simulink model "TEST"  (R2021a)
settings: Solver=VariableStepAuto  StartTime=0.0  StopTime=10  RelTol=1e-3
undefined symbols (not defined in the file): f, Jw, Kb, Kt, La, Ra
libraries: vrlib x1
settings Model: Creator=mario  LastModifiedBy=mario
settings SolverCC: AlgebraicLoopSolver=TrustRegion
settings DataIOCC: ReturnWorkspaceOutputs=off
settings DebuggingCC: SFMachineParentedDataDiag=warning  ArithmeticOperatorsInVariantConditions=warning
settings SFSimCC: CustomCodeUndefinedFunction=UseInterfaceOnly

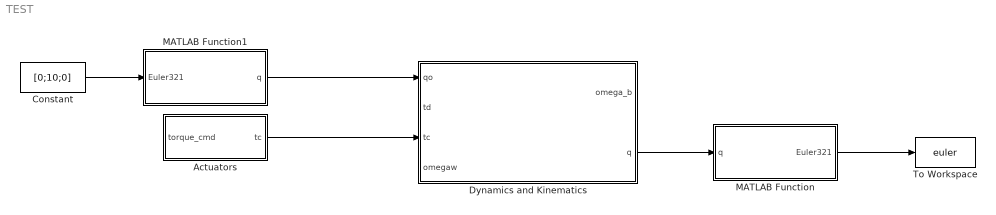
== system TEST ==
  Actuators : Subsystem
  Constant : Constant  Value=[0;10;0]
  "Dynamics and Kinematics " : Subsystem
  MATLAB Function : MATLAB Function  TreatAsAtomicUnit=on
  MATLAB Function1 : MATLAB Function  TreatAsAtomicUnit=on
  To Workspace : ToWorkspace  VariableName=euler  SampleTime=0.05
  wires:
  "Dynamics and Kinematics "/2(q) -> MATLAB Function/1(q)
  MATLAB Function/1(Euler321) -> To Workspace/1
  MATLAB Function1/1(q) -> "Dynamics and Kinematics "/1(qo)
  Constant/1 -> MATLAB Function1/1(Euler321)
  Actuators/1(tc) -> "Dynamics and Kinematics "/3(tc)

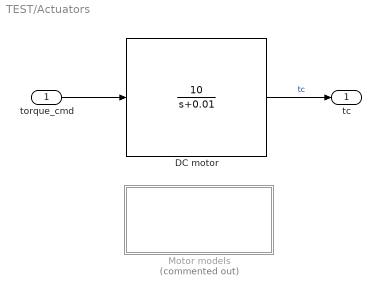
== system TEST/Actuators ==
  torque_cmd : Inport
  DC motor : TransferFcn  Numerator=[10]  Denominator=[1 0.01 ]
  Motor models : Subsystem  Commented=on
  tc : Outport
  wires:
  torque_cmd/1 -> DC motor/1
  DC motor/1 -> tc/1  "tc"

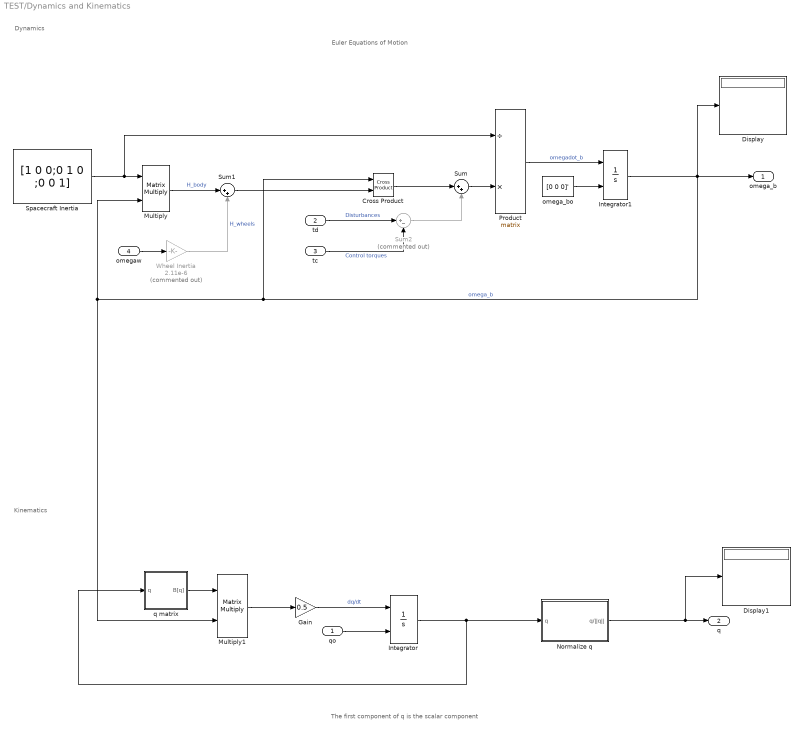
== system TEST/Dynamics and Kinematics  ==
  note: The first component of q is the scalar component
  note: Euler Equations of Motion
  note: Dynamics
  note: Kinematics
  qo : Inport
  td : Inport  Port=2
  tc : Inport  Port=3
  omegaw : Inport  Port=4
  Cross Product : vrlib/Utilities/Cross Product
  Display : Display
  Display1 : Display
  Gain : Gain  Gain=0.5
  Integrator : Integrator  InitialConditionSource=external
  Integrator1 : Integrator  InitialConditionSource=external
  Multiply : Product  Multiplication=Matrix(*)
  Multiply1 : Product  Multiplication=Matrix(*)
  Normalize q : Subsystem
  Product : Product  Inputs=/*  Multiplication=Matrix(*)
  Spacecraft Inertia : Constant  Value=[1 0 0;0 1 0 ;0 0 1]
  Sum : Sum  Inputs=|++
  Sum1 : Sum  Inputs=|++
  Sum2 : Sum  Commented=on  Inputs=|+-
  Wheel Inertia : Gain  Commented=on  Gain=2.11e-6
  omega_bo : Constant  Value=[0 0 0]'
  q matrix : Subsystem
  omega_b : Outport  VectorParamsAs1DForOutWhenUnconnected=off
  q : Outport  Port=2  VectorParamsAs1DForOutWhenUnconnected=off
  wires:
  q matrix/1(B[q]) -> Multiply1/1
  Integrator/1 -> q matrix/1(q), Normalize q/1(q)
  Gain/1 -> Integrator/1  "dq/dt"
  Multiply1/1 -> Gain/1
  Sum2/1 -> Sum/2
  Wheel Inertia/1 -> Sum1/2  "H_wheels"
  Sum1/1 -> Cross Product/2
  Cross Product/1 -> Sum/1
  Sum/1 -> Product/2
  Multiply/1 -> Sum1/1  "H_body"
  Product/1 -> Integrator1/1  "omegadot_b"
  omega_bo/1 -> Integrator1/2
  Spacecraft Inertia/1 -> Multiply/1, Product/1
  Integrator1/1 -> omega_b/1, Display/1, Multiply1/2, Multiply/2, Cross Product/1  "omega_b"
  Normalize q/1(q/||q||) -> Display1/1, q/1
  qo/1 -> Integrator/2
  td/1 -> Sum2/1  "Disturbances"
  tc/1 -> Sum2/2  "Control torques"
  omegaw/1 -> Wheel Inertia/1

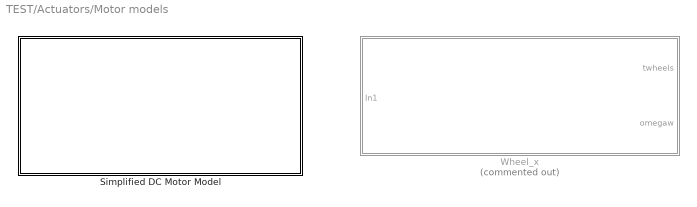
== system TEST/Actuators/Motor models ==
  Simplified DC Motor Model : Subsystem
  Wheel_x : Subsystem  Commented=on

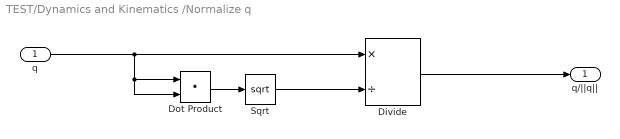
== system TEST/Dynamics and Kinematics /Normalize q ==
  q : Inport
  Divide : Product  Inputs=*/
  Dot Product : DotProduct  InputSameDT=on  OutDataTypeStr=Inherit: Inherit via internal rule
  Sqrt : Sqrt  SaturateOnIntegerOverflow=on
  q/||q|| : Outport  VectorParamsAs1DForOutWhenUnconnected=off
  wires:
  Divide/1 -> q/||q||/1
  Dot Product/1 -> Sqrt/1
  Sqrt/1 -> Divide/2
  q/1 -> Dot Product/1, Dot Product/2, Divide/1

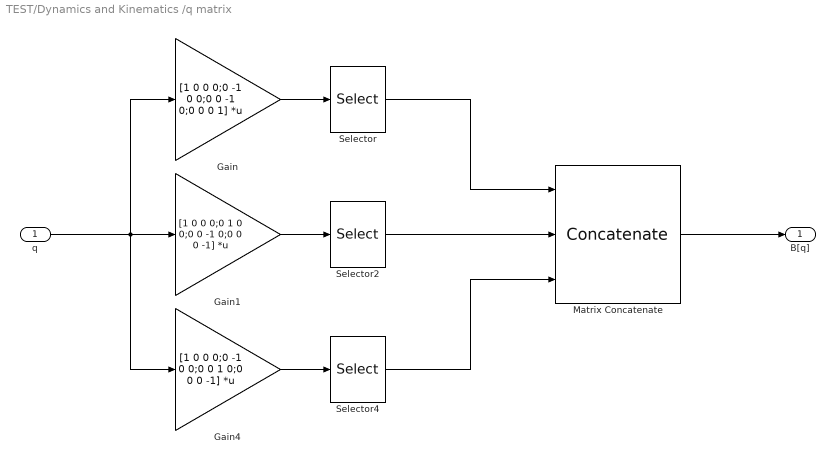
== system TEST/Dynamics and Kinematics /q matrix ==
  q : Inport
  Gain : Gain  Gain=[1 0 0 0;0 -1 0 0;0 0 -1 0;0 0 0 1]  Multiplication=Matrix(K*u)
  Gain1 : Gain  Gain=[1 0 0 0;0 1 0 0;0 0 -1 0;0 0 0 -1]  Multiplication=Matrix(K*u)
  Gain4 : Gain  Gain=[1 0 0 0;0 -1 0 0;0 0 1 0;0 0 0 -1]  Multiplication=Matrix(K*u)
  Matrix Concatenate : Concatenate  NumInputs=3  Mode=Multidimensional array  ConcatenateDimension=2
  Selector : Selector  InputPortWidth=4  IndexOptions=Index vector (dialog)  Indices=[2 1 4 3]  OutputSizes=1
  Selector2 : Selector  InputPortWidth=4  IndexOptions=Index vector (dialog)  Indices=[3 4 1 2]  OutputSizes=1
  Selector4 : Selector  InputPortWidth=4  IndexOptions=Index vector (dialog)  Indices=[4 3 2 1]  OutputSizes=1
  B[q] : Outport  VectorParamsAs1DForOutWhenUnconnected=off
  wires:
  Gain/1 -> Selector/1
  Gain1/1 -> Selector2/1
  Selector/1 -> Matrix Concatenate/1
  q/1 -> Gain1/1, Gain/1, Gain4/1
  Selector4/1 -> Matrix Concatenate/3
  Matrix Concatenate/1 -> B[q]/1
  Selector2/1 -> Matrix Concatenate/2
  Gain4/1 -> Selector4/1

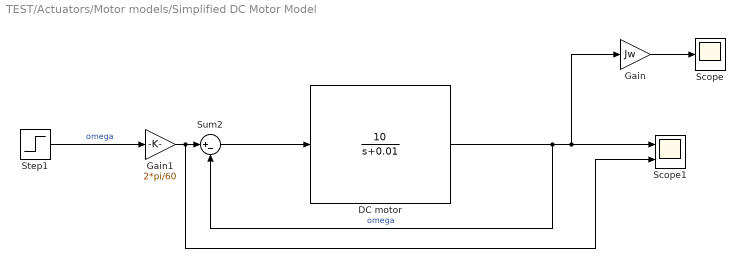
== system TEST/Actuators/Motor models/Simplified DC Motor Model ==
  DC motor : TransferFcn  Numerator=[10]  Denominator=[1 0.01 ]
  Gain : Gain  Gain=Jw
  Gain1 : Gain  Gain=2*pi/60
  Scope : Scope
  Scope1 : Scope  NumInputPorts=2
  Step1 : Step  Time=0  After=8000  SampleTime=0
  Sum2 : Sum  Inputs=|+-
  wires:
  Step1/1 -> Gain1/1  "omega"
  Sum2/1 -> DC motor/1
  DC motor/1 -> Gain/1, Scope1/1, Sum2/2  "omega"
  Gain1/1 -> Scope1/2, Sum2/1
  Gain/1 -> Scope/1

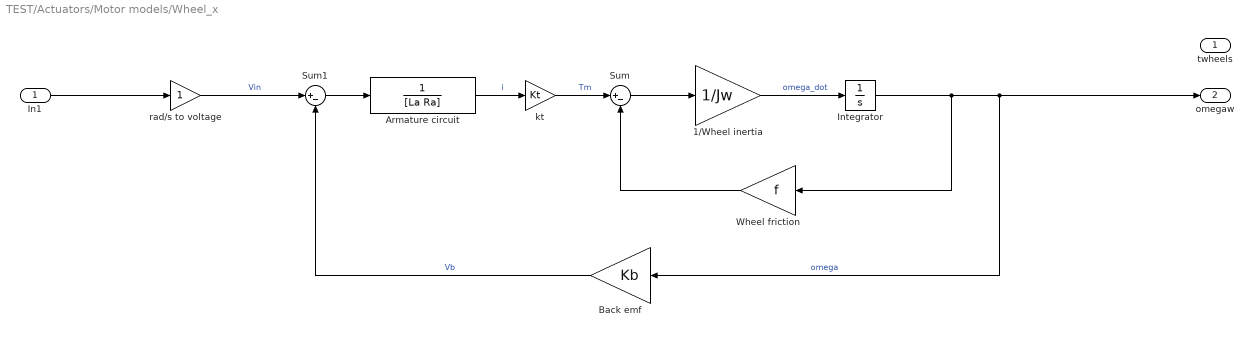
== system TEST/Actuators/Motor models/Wheel_x ==
  In1 : Inport
  1/Wheel inertia : Gain  Gain=1/Jw
  Armature circuit : TransferFcn  Denominator=[La Ra]
  Back emf : Gain  Gain=Kb
  Integrator : Integrator
  Sum : Sum  Inputs=|+-
  Sum1 : Sum  Inputs=|+-
  Wheel friction : Gain  Gain=f
  kt : Gain  Gain=Kt
  rad/s to voltage : Gain
  twheels : Outport  VectorParamsAs1DForOutWhenUnconnected=off
  omegaw : Outport  Port=2  VectorParamsAs1DForOutWhenUnconnected=off
  wires:
  rad/s to voltage/1 -> Sum1/1  "Vin"
  Back emf/1 -> Sum1/2  "Vb"
  Sum/1 -> 1/Wheel inertia/1
  kt/1 -> Sum/1  "Tm"
  1/Wheel inertia/1 -> Integrator/1  "omega_dot"
  Sum1/1 -> Armature circuit/1
  Wheel friction/1 -> Sum/2
  Integrator/1 -> Wheel friction/1, omegaw/1, Back emf/1  "omega"
  Armature circuit/1 -> kt/1  "i"
  In1/1 -> rad/s to voltage/1

== matlab function TEST/MATLAB Function ==
  data: q input; Euler321 output
function Euler321 = q2euler(q)
q1 = q(1);
qbar = [q(2);q(3);q(4)];
qtilde = [0 -qbar(3) qbar(2);qbar(3) 0 -qbar(1);-qbar(2) qbar(1) 0];

DCM = 2*(qbar*qbar') + (q1^2-qbar'*qbar)*eye(3) - 2*q1*qtilde;

Euler321 = [atan2(DCM(1,2),DCM(1,1));-asin(DCM(1,3)); atan2(DCM(2,3),DCM(3,3))];

== matlab function TEST/MATLAB Function1 ==
  data: Euler321 input; q output
function q = euler3212q(Euler321)
euler = [deg2rad(Euler321(1));deg2rad(Euler321(2));deg2rad(Euler321(3))];

c1 = cos(euler(1)/2);
s1 = sin(euler(1)/2);
c2 = cos(euler(2)/2);
s2 = sin(euler(2)/2);
c3 = cos(euler(3)/2);
s3 = sin(euler(3)/2);

q = [c1*c2*c3+s1*s2*s3 ;
     s1*c2*c3-c1*s2*s3;
     c1*s2*c3+s1*c2*s3;
     c1*c2*s3-s1*s2*c3];
